simulink model "CarSpeedControllerTest2"  (R2023b)
settings: Solver=VariableStepAuto  StartTime=0.0  StopTime=600  RelTol=1e-3
libraries: slpidlib x2
settings Model: Creator=fiona  LastModifiedBy=fiona

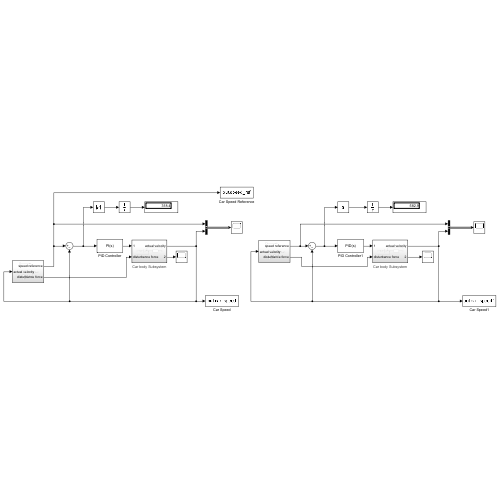
[thumbnail: Simulink's stored preview of the top-level diagram]
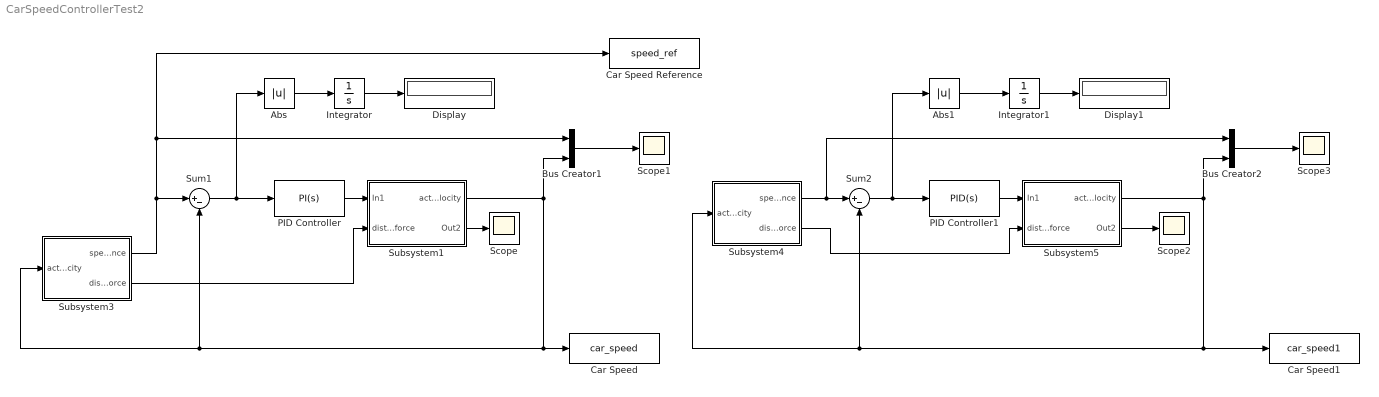
== system CarSpeedControllerTest2 ==
  Abs : Abs  SaturateOnIntegerOverflow=off
  Abs1 : Abs  SaturateOnIntegerOverflow=off
  Bus Creator1 : BusCreator  Inputs=2
  Bus Creator2 : BusCreator  Inputs=2
  Car Speed : ToWorkspace  VariableName=car_speed  SaveFormat=Timeseries  SampleTime=-1
  Car Speed Reference : ToWorkspace  VariableName=speed_ref  SaveFormat=Timeseries  SampleTime=-1
  Car Speed1 : ToWorkspace  VariableName=car_speed1  SaveFormat=Timeseries  SampleTime=-1
  Display : Display
  Display1 : Display
  Integrator : Integrator
  Integrator1 : Integrator
  PID Controller : slpidlib/PID Controller  Controller=PI  Form=Parallel  TimeDomain=Continuous-time  UseExternalTs=off  SampleTime=-1  IntegratorMethod=Forward Euler  FilterMethod=Forward Euler  ControllerParametersSource=internal  P=22.6  I=3.57  UseKiTs=off  D=1  N=100  UseFilter=on  TunerSelectOption=Transfer Function Based (PID Tuner App)  InitialConditionSource=internal  InitialConditionForIntegrator=0  InitialConditionForFilter=0  DifferentiatorICPrevScaledInput=0  ExternalReset=none  TrackingMode=off  Kt=1  LimitOutput=off  SatLimitsSource=internal  UpperSaturationLimit=inf  LowerSaturationLimit=-inf  LinearizeAsGain=on  AntiWindupMode=none  Kb=1  LimitIntegrator=off  UpperIntegratorSaturationLimit=inf  LowerIntegratorSaturationLimit=-inf  POutMin=[]  POutMax=[]  IOutMin=[]  IOutMax=[]  DOutMin=[]  DOutMax=[]  NOutMin=[]  NOutMax=[]  SumOutMin=[]  SumOutMax=[]  SaturationOutMin=[]  SaturationOutMax=[]  PParamMin=[]  PParamMax=[]  IParamMin=[]  IParamMax=[]  DParamMin=[]  DParamMax=[]  NParamMin=[]  NParamMax=[]  KbParamMin=[]  KbParamMax=[]  KtParamMin=[]  KtParamMax=[]  KbOutMin=[]  KbOutMax=[]  KtOutMin=[]  KtOutMax=[]  IntegratorOutMin=[]  IntegratorOutMax=[]  FilterOutMin=[]  FilterOutMax=[]  SumI1OutMin=[]  SumI1OutMax=[]  SumI2OutMin=[]  SumI2OutMax=[]  SumI3OutMin=[]  SumI3OutMax=[]  SumI4OutMin=[]  SumI4OutMax=[]  SumDOutMin=[]  SumDOutMax=[]  DifferentiatorOutMin=[]  DifferentiatorOutMax=[]  FilterDiffOutCoefMin=[]  FilterDiffOutCoefMax=[]  ReciprocalOutMin=[]  ReciprocalOutMax=[]  SumDenOutMin=[]  SumDenOutMax=[]  SumNumOutMin=[]  SumNumOutMax=[]  DivideOutMin=[]  DivideOutMax=[]  UdiffTsProdOutMin=[]  UdiffTsProdOutMax=[]  NTsProdOutMin=[]  NTsProdOutMax=[]  UintegralTsProdOutMin=[]  UintegralTsProdOutMax=[]  UngainTsProdOutMin=[]  UngainTsProdOutMax=[]  ClampingZeroOutDataTypeStr=Inherit: Inherit via back propagation  ClampingZeroOutMin=[]  ClampingZeroOutMax=[]  FilterDenConstantOutDataTypeStr=Inherit: Inherit via back propagation  FilterDenConstantOutMin=[]  FilterDenConstantOutMax=[]  PCopyOutDataTypeStr=Inherit: Inherit via back propagation  PCopyOutMin=[]  PCopyOutMax=[]  NCopyOutDataTypeStr=Inherit: Inherit via back propagation  NCopyOutMin=[]  NCopyOutMax=[]  IntegratorContinuousStateAttributes=''  IntegratorStateMustResolveToSignalObject=off  IntegratorRTWStateStorageClass=Auto  FilterContinuousStateAttributes=''  FilterStateMustResolveToSignalObject=off  FilterRTWStateStorageClass=Auto  ParallelPVariant=InternalParameters  IdealPVariant=Disabled  IVariant=InternalParameters  DVariant=Disabled  IntegratorVariant=Continuous  SatVariant=Disabled  AWVariant=Passthrough  PCopyVariant=Disabled  TRVariant=Disabled  FdbkBlocksVariant=Forward  IdealPFdbkVariant=Disabled  SatFdbkVariant=Disabled  DerivativeFilterVariant=Disabled  NVariant=Disabled  NCopyVariant=Disabled_SignalSpec  FilterICVariant=Disabled  IntegratorICVariant=InternalICs  ExternalResetVariant=Disabled  TRSumVariant=Passthrough  SumFdbkVariant=Disabled  SumVariant=Sum_PI  TsampFilterVariant=InternalTs  TsampNgainVariant=Passthrough  TsampIntegralVariant=Disabled_SignalSpec  ExternalSaturationOutDataTypeStr=Inherit: Same as second input
  PID Controller1 : slpidlib/PID Controller  Controller=PID  Form=Parallel  TimeDomain=Continuous-time  UseExternalTs=off  SampleTime=-1  IntegratorMethod=Forward Euler  FilterMethod=Forward Euler  ControllerParametersSource=internal  P=37  I=0.964  UseKiTs=off  D=10.9  N=2.5  UseFilter=on  TunerSelectOption=Transfer Function Based (PID Tuner App)  InitialConditionSource=internal  InitialConditionForIntegrator=0  InitialConditionForFilter=0  DifferentiatorICPrevScaledInput=0  ExternalReset=none  TrackingMode=off  Kt=1  LimitOutput=off  SatLimitsSource=internal  UpperSaturationLimit=inf  LowerSaturationLimit=-inf  LinearizeAsGain=on  AntiWindupMode=none  Kb=1  LimitIntegrator=off  UpperIntegratorSaturationLimit=inf  LowerIntegratorSaturationLimit=-inf  POutMin=[]  POutMax=[]  IOutMin=[]  IOutMax=[]  DOutMin=[]  DOutMax=[]  NOutMin=[]  NOutMax=[]  SumOutMin=[]  SumOutMax=[]  SaturationOutMin=[]  SaturationOutMax=[]  PParamMin=[]  PParamMax=[]  IParamMin=[]  IParamMax=[]  DParamMin=[]  DParamMax=[]  NParamMin=[]  NParamMax=[]  KbParamMin=[]  KbParamMax=[]  KtParamMin=[]  KtParamMax=[]  KbOutMin=[]  KbOutMax=[]  KtOutMin=[]  KtOutMax=[]  IntegratorOutMin=[]  IntegratorOutMax=[]  FilterOutMin=[]  FilterOutMax=[]  SumI1OutMin=[]  SumI1OutMax=[]  SumI2OutMin=[]  SumI2OutMax=[]  SumI3OutMin=[]  SumI3OutMax=[]  SumI4OutMin=[]  SumI4OutMax=[]  SumDOutMin=[]  SumDOutMax=[]  DifferentiatorOutMin=[]  DifferentiatorOutMax=[]  FilterDiffOutCoefMin=[]  FilterDiffOutCoefMax=[]  ReciprocalOutMin=[]  ReciprocalOutMax=[]  SumDenOutMin=[]  SumDenOutMax=[]  SumNumOutMin=[]  SumNumOutMax=[]  DivideOutMin=[]  DivideOutMax=[]  UdiffTsProdOutMin=[]  UdiffTsProdOutMax=[]  NTsProdOutMin=[]  NTsProdOutMax=[]  UintegralTsProdOutMin=[]  UintegralTsProdOutMax=[]  UngainTsProdOutMin=[]  UngainTsProdOutMax=[]  ClampingZeroOutDataTypeStr=Inherit: Inherit via back propagation  ClampingZeroOutMin=[]  ClampingZeroOutMax=[]  FilterDenConstantOutDataTypeStr=Inherit: Inherit via back propagation  FilterDenConstantOutMin=[]  FilterDenConstantOutMax=[]  PCopyOutDataTypeStr=Inherit: Inherit via back propagation  PCopyOutMin=[]  PCopyOutMax=[]  NCopyOutDataTypeStr=Inherit: Inherit via back propagation  NCopyOutMin=[]  NCopyOutMax=[]  IntegratorContinuousStateAttributes=''  IntegratorStateMustResolveToSignalObject=off  IntegratorRTWStateStorageClass=Auto  FilterContinuousStateAttributes=''  FilterStateMustResolveToSignalObject=off  FilterRTWStateStorageClass=Auto  ParallelPVariant=InternalParameters  IdealPVariant=Disabled  IVariant=InternalParameters  DVariant=InternalParameters  IntegratorVariant=Continuous  SatVariant=Disabled  AWVariant=Passthrough  PCopyVariant=Disabled  TRVariant=Disabled  FdbkBlocksVariant=Forward  IdealPFdbkVariant=Disabled  SatFdbkVariant=Disabled  DerivativeFilterVariant=ContFilter  NVariant=InternalParameters  NCopyVariant=Disabled  FilterICVariant=InternalICsFilter  IntegratorICVariant=InternalICs  ExternalResetVariant=Disabled  TRSumVariant=Passthrough  SumFdbkVariant=Disabled  SumVariant=Sum_PID  TsampFilterVariant=InternalTs  TsampNgainVariant=Passthrough  TsampIntegralVariant=Disabled_SignalSpec  ExternalSaturationOutDataTypeStr=Inherit: Same as second input
  Scope{,1..3} (4 alike) : Scope
  Subsystem1 : Subsystem
      settings: AttributesFormatString=Car body Subsystem
  Subsystem3 : Subsystem
  Subsystem4 : Subsystem
  Subsystem5 : Subsystem
      settings: AttributesFormatString=Car body Subsystem
  Sum1 : Sum  Inputs=|+-
  Sum2 : Sum  Inputs=|+-
  wires:
  Subsystem3/1(speed reference) -> Car Speed Reference/1, Bus Creator1/1, Sum1/1
  Subsystem1/1(actual velocity) -> Subsystem3/1(actual velocity), Sum1/2, Car Speed/1, Bus Creator1/2
  Bus Creator1/1 -> Scope1/1
  Subsystem1/2(Out2) -> Scope/1
  Subsystem3/2(disturbance force) -> Subsystem1/2(disturbance force)
  Subsystem5/1(actual velocity) -> Bus Creator2/2, Sum2/2, Subsystem4/1(actual velocity), Car Speed1/1
  Bus Creator2/1 -> Scope3/1
  PID Controller/1 -> Subsystem1/1(In1)
  Sum1/1 -> Abs/1, PID Controller/1
  Abs/1 -> Integrator/1
  Integrator/1 -> Display/1
  Integrator1/1 -> Display1/1
  Abs1/1 -> Integrator1/1
  PID Controller1/1 -> Subsystem5/1(In1)
  Sum2/1 -> PID Controller1/1, Abs1/1
  Subsystem4/1(speed reference) -> Bus Creator2/1, Sum2/1
  Subsystem4/2(disturbance force) -> Subsystem5/2(disturbance force)
  Subsystem5/2(Out2) -> Scope2/1

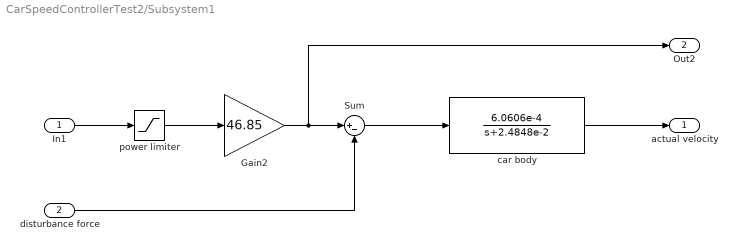
== system CarSpeedControllerTest2/Subsystem1 ==
  In1 : Inport
  disturbance force : Inport  Port=2
  Gain2 : Gain  Gain=46.85
  Sum : Sum  Inputs=|+-
  car body : TransferFcn  Numerator=[6.0606e-4]  Denominator=[1 2.4848e-2]  ContinuousStateAttributes='position'
  power limiter : Saturate  UpperLimit=1921  LowerLimit=-1921
  actual velocity : Outport
  Out2 : Outport  Port=2
  wires:
  Sum/1 -> car body/1
  In1/1 -> power limiter/1
  car body/1 -> actual velocity/1
  disturbance force/1 -> Sum/2
  power limiter/1 -> Gain2/1
  Gain2/1 -> Out2/1, Sum/1

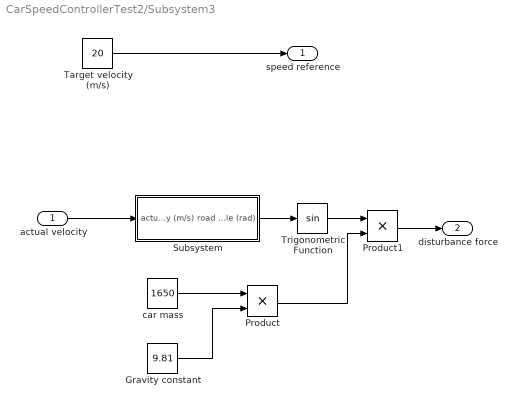
== system CarSpeedControllerTest2/Subsystem3 ==
  actual velocity : Inport
  Gravity constant : Constant  Value=9.81
  Product : Product
  Product1 : Product
  Subsystem : Subsystem
  Target velocity (m/s) : Constant  Value=20
  Trigonometric Function : Trigonometry
  car mass : Constant  Value=1650
  speed reference : Outport
  disturbance force : Outport  Port=2
  wires:
  actual velocity/1 -> Subsystem/1(actual velocity (m/s))
  Subsystem/1(road slope angle (rad)) -> Trigonometric Function/1
  Target velocity (m/s)/1 -> speed reference/1
  Trigonometric Function/1 -> Product1/1
  Product/1 -> Product1/2
  car mass/1 -> Product/1
  Gravity constant/1 -> Product/2
  Product1/1 -> disturbance force/1

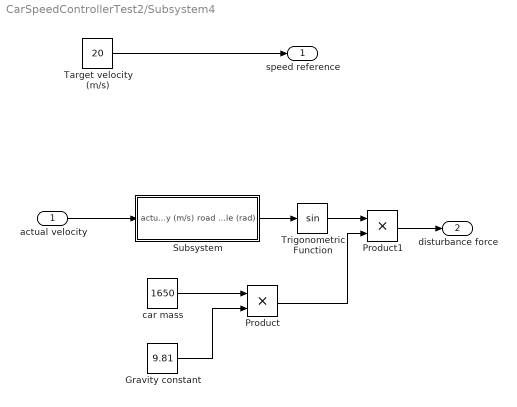
== system CarSpeedControllerTest2/Subsystem4 ==
  actual velocity : Inport
  Gravity constant : Constant  Value=9.81
  Product : Product
  Product1 : Product
  Subsystem : Subsystem
  Target velocity (m/s) : Constant  Value=20
  Trigonometric Function : Trigonometry
  car mass : Constant  Value=1650
  speed reference : Outport
  disturbance force : Outport  Port=2
  wires:
  actual velocity/1 -> Subsystem/1(actual velocity (m/s))
  Subsystem/1(road slope angle (rad)) -> Trigonometric Function/1
  Target velocity (m/s)/1 -> speed reference/1
  Trigonometric Function/1 -> Product1/1
  Product/1 -> Product1/2
  car mass/1 -> Product/1
  Gravity constant/1 -> Product/2
  Product1/1 -> disturbance force/1

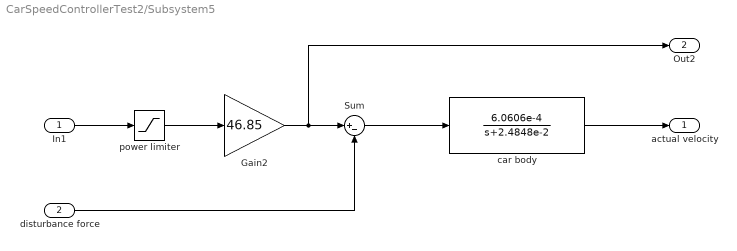
== system CarSpeedControllerTest2/Subsystem5 ==
  In1 : Inport
  disturbance force : Inport  Port=2
  Gain2 : Gain  Gain=46.85
  Sum : Sum  Inputs=|+-
  car body : TransferFcn  Numerator=[6.0606e-4]  Denominator=[1 2.4848e-2]  ContinuousStateAttributes='position'
  power limiter : Saturate  UpperLimit=1921  LowerLimit=-1921
  actual velocity : Outport
  Out2 : Outport  Port=2
  wires:
  Sum/1 -> car body/1
  In1/1 -> power limiter/1
  car body/1 -> actual velocity/1
  disturbance force/1 -> Sum/2
  power limiter/1 -> Gain2/1
  Gain2/1 -> Out2/1, Sum/1

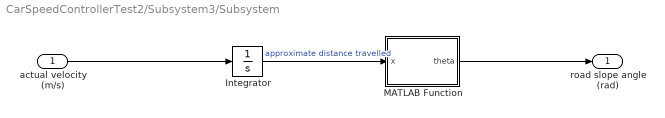
== system CarSpeedControllerTest2/Subsystem3/Subsystem ==
  actual velocity (m/s) : Inport
  Integrator : Integrator
  MATLAB Function : MATLAB Function  TreatAsAtomicUnit=on
  road slope angle (rad) : Outport
  wires:
  MATLAB Function/1(theta) -> road slope angle (rad)/1
  actual velocity (m/s)/1 -> Integrator/1
  Integrator/1 -> MATLAB Function/1(x)  "approximate distance travelled"

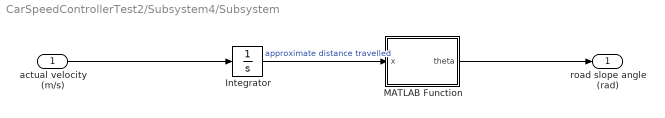
== system CarSpeedControllerTest2/Subsystem4/Subsystem ==
  actual velocity (m/s) : Inport
  Integrator : Integrator
  MATLAB Function : MATLAB Function  TreatAsAtomicUnit=on
  road slope angle (rad) : Outport
  wires:
  MATLAB Function/1(theta) -> road slope angle (rad)/1
  actual velocity (m/s)/1 -> Integrator/1
  Integrator/1 -> MATLAB Function/1(x)  "approximate distance travelled"

== matlab function CarSpeedControllerTest2/Subsystem3/Subsystem/MATLAB Function ==
  data: x input; theta output
function theta = fcn(x)

theta = pi/18*exp(0.0001*x)*sin(0.0015*x)*cos(0.001*x)+pi/18;

== matlab function CarSpeedControllerTest2/Subsystem4/Subsystem/MATLAB Function ==
  data: x input; theta output
function theta = fcn(x)

theta = pi/18*exp(0.0001*x)*sin(0.0015*x)*cos(0.001*x)+pi/18;
